simulink model "xEMU_SimulationModel3_rule1"  (R2017b)
settings: Solver=ode4  StartTime=0.0  StopTime=8192  FixedStep=0.01  RelTol=1e-3
undefined symbols (not defined in the file): a1, a2, a3, a4, ACO, BAT, Battery, DCT, DRT, EMS, ENV, Fahrzyklus_VS_modell, height_BAT, leistung, lib_bat, Maximum, Maximum_position, Num_cells, P_FC_max_long, P_FC_min_long, P_FC_step_max, Pbat_charge_max, Pbat_discharge_max, Pfc_max, Pfc_min, SOC_tar, time_peaks, TRM, velocity_peaks
libraries: simulink x5
(part 8 of 15)

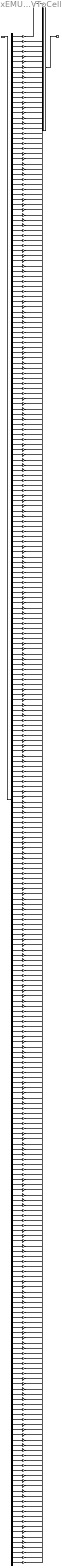
== system xEMU_SimulationModel3_rule1/Battery (BAT)_mittel_02/Cell/Thermal/FVToCell ==
  T_FV : Inport
  AddCell1 : Sum  Inputs=<binary blob, 300 chars, not shown>
  Demux : Demux  Outputs=300
  T_FV_{1..300} (300 alike) : Gain  Gain=0.0033333  SaturateOnIntegerOverflow=on  OutDataTypeStr=Inherit: Same as input  ParamDataTypeStr=Inherit: Same as input
  tag scope: T_CellElement1=global
  wires:
  T_FV/1 -> Demux/1
  Demux/1 -> T_FV_1/1
  Demux/2 -> T_FV_2/1
  Demux/3 -> T_FV_3/1
  Demux/4 -> T_FV_4/1
  Demux/5 -> T_FV_5/1
  Demux/6 -> T_FV_6/1
  Demux/7 -> T_FV_7/1
  Demux/8 -> T_FV_8/1
  Demux/9 -> T_FV_9/1
  Demux/10 -> T_FV_10/1
  Demux/11 -> T_FV_11/1
  Demux/12 -> T_FV_12/1
  Demux/13 -> T_FV_13/1
  Demux/14 -> T_FV_14/1
  Demux/15 -> T_FV_15/1
  Demux/16 -> T_FV_16/1
  Demux/17 -> T_FV_17/1
  Demux/18 -> T_FV_18/1
  Demux/19 -> T_FV_19/1
  Demux/20 -> T_FV_20/1
  Demux/21 -> T_FV_21/1
  Demux/22 -> T_FV_22/1
  Demux/23 -> T_FV_23/1
  Demux/24 -> T_FV_24/1
  Demux/25 -> T_FV_25/1
  Demux/26 -> T_FV_26/1
  Demux/27 -> T_FV_27/1
  Demux/28 -> T_FV_28/1
  Demux/29 -> T_FV_29/1
  Demux/30 -> T_FV_30/1
  Demux/31 -> T_FV_31/1
  Demux/32 -> T_FV_32/1
  Demux/33 -> T_FV_33/1
  Demux/34 -> T_FV_34/1
  Demux/35 -> T_FV_35/1
  Demux/36 -> T_FV_36/1
  Demux/37 -> T_FV_37/1
  Demux/38 -> T_FV_38/1
  Demux/39 -> T_FV_39/1
  Demux/40 -> T_FV_40/1
  Demux/41 -> T_FV_41/1
  Demux/42 -> T_FV_42/1
  Demux/43 -> T_FV_43/1
  Demux/44 -> T_FV_44/1
  Demux/45 -> T_FV_45/1
  Demux/46 -> T_FV_46/1
  Demux/47 -> T_FV_47/1
  Demux/48 -> T_FV_48/1
  Demux/49 -> T_FV_49/1
  Demux/50 -> T_FV_50/1
  Demux/51 -> T_FV_51/1
  Demux/52 -> T_FV_52/1
  Demux/53 -> T_FV_53/1
  Demux/54 -> T_FV_54/1
  Demux/55 -> T_FV_55/1
  Demux/56 -> T_FV_56/1
  Demux/57 -> T_FV_57/1
  Demux/58 -> T_FV_58/1
  Demux/59 -> T_FV_59/1
  Demux/60 -> T_FV_60/1
  Demux/61 -> T_FV_61/1
  Demux/62 -> T_FV_62/1
  Demux/63 -> T_FV_63/1
  Demux/64 -> T_FV_64/1
  Demux/65 -> T_FV_65/1
  Demux/66 -> T_FV_66/1
  Demux/67 -> T_FV_67/1
  Demux/68 -> T_FV_68/1
  Demux/69 -> T_FV_69/1
  Demux/70 -> T_FV_70/1
  Demux/71 -> T_FV_71/1
  Demux/72 -> T_FV_72/1
  Demux/73 -> T_FV_73/1
  Demux/74 -> T_FV_74/1
  Demux/75 -> T_FV_75/1
  Demux/76 -> T_FV_76/1
  Demux/77 -> T_FV_77/1
  Demux/78 -> T_FV_78/1
  Demux/79 -> T_FV_79/1
  Demux/80 -> T_FV_80/1
  Demux/81 -> T_FV_81/1
  Demux/82 -> T_FV_82/1
  Demux/83 -> T_FV_83/1
  Demux/84 -> T_FV_84/1
  Demux/85 -> T_FV_85/1
  Demux/86 -> T_FV_86/1
  Demux/87 -> T_FV_87/1
  Demux/88 -> T_FV_88/1
  Demux/89 -> T_FV_89/1
  Demux/90 -> T_FV_90/1
  Demux/91 -> T_FV_91/1
  Demux/92 -> T_FV_92/1
  Demux/93 -> T_FV_93/1
  Demux/94 -> T_FV_94/1
  Demux/95 -> T_FV_95/1
  Demux/96 -> T_FV_96/1
  Demux/97 -> T_FV_97/1
  Demux/98 -> T_FV_98/1
  Demux/99 -> T_FV_99/1
  Demux/100 -> T_FV_100/1
  Demux/101 -> T_FV_101/1
  Demux/102 -> T_FV_102/1
  Demux/103 -> T_FV_103/1
  Demux/104 -> T_FV_104/1
  Demux/105 -> T_FV_105/1
  Demux/106 -> T_FV_106/1
  Demux/107 -> T_FV_107/1
  Demux/108 -> T_FV_108/1
  Demux/109 -> T_FV_109/1
  Demux/110 -> T_FV_110/1
  Demux/111 -> T_FV_111/1
  Demux/112 -> T_FV_112/1
  Demux/113 -> T_FV_113/1
  Demux/114 -> T_FV_114/1
  Demux/115 -> T_FV_115/1
  Demux/116 -> T_FV_116/1
  Demux/117 -> T_FV_117/1
  Demux/118 -> T_FV_118/1
  Demux/119 -> T_FV_119/1
  Demux/120 -> T_FV_120/1
  Demux/121 -> T_FV_121/1
  Demux/122 -> T_FV_122/1
  Demux/123 -> T_FV_123/1
  Demux/124 -> T_FV_124/1
  Demux/125 -> T_FV_125/1
  Demux/126 -> T_FV_126/1
  Demux/127 -> T_FV_127/1
  Demux/128 -> T_FV_128/1
  Demux/129 -> T_FV_129/1
  Demux/130 -> T_FV_130/1
  Demux/131 -> T_FV_131/1
  Demux/132 -> T_FV_132/1
  Demux/133 -> T_FV_133/1
  Demux/134 -> T_FV_134/1
  Demux/135 -> T_FV_135/1
  Demux/136 -> T_FV_136/1
  Demux/137 -> T_FV_137/1
  Demux/138 -> T_FV_138/1
  Demux/139 -> T_FV_139/1
  Demux/140 -> T_FV_140/1
  Demux/141 -> T_FV_141/1
  Demux/142 -> T_FV_142/1
  Demux/143 -> T_FV_143/1
  Demux/144 -> T_FV_144/1
  Demux/145 -> T_FV_145/1
  Demux/146 -> T_FV_146/1
  Demux/147 -> T_FV_147/1
  Demux/148 -> T_FV_148/1
  Demux/149 -> T_FV_149/1
  Demux/150 -> T_FV_150/1
  Demux/151 -> T_FV_151/1
  Demux/152 -> T_FV_152/1
  Demux/153 -> T_FV_153/1
  Demux/154 -> T_FV_154/1
  Demux/155 -> T_FV_155/1
  Demux/156 -> T_FV_156/1
  Demux/157 -> T_FV_157/1
  Demux/158 -> T_FV_158/1
  Demux/159 -> T_FV_159/1
  Demux/160 -> T_FV_160/1
  Demux/161 -> T_FV_161/1
  Demux/162 -> T_FV_162/1
  Demux/163 -> T_FV_163/1
  Demux/164 -> T_FV_164/1
  Demux/165 -> T_FV_165/1
  Demux/166 -> T_FV_166/1
  Demux/167 -> T_FV_167/1
  Demux/168 -> T_FV_168/1
  Demux/169 -> T_FV_169/1
  Demux/170 -> T_FV_170/1
  Demux/171 -> T_FV_171/1
  Demux/172 -> T_FV_172/1
  Demux/173 -> T_FV_173/1
  Demux/174 -> T_FV_174/1
  Demux/175 -> T_FV_175/1
  Demux/176 -> T_FV_176/1
  Demux/177 -> T_FV_177/1
  Demux/178 -> T_FV_178/1
  Demux/179 -> T_FV_179/1
  Demux/180 -> T_FV_180/1
  Demux/181 -> T_FV_181/1
  Demux/182 -> T_FV_182/1
  Demux/183 -> T_FV_183/1
  Demux/184 -> T_FV_184/1
  Demux/185 -> T_FV_185/1
  Demux/186 -> T_FV_186/1
  Demux/187 -> T_FV_187/1
  Demux/188 -> T_FV_188/1
  Demux/189 -> T_FV_189/1
  Demux/190 -> T_FV_190/1
  Demux/191 -> T_FV_191/1
  Demux/192 -> T_FV_192/1
  Demux/193 -> T_FV_193/1
  Demux/194 -> T_FV_194/1
  Demux/195 -> T_FV_195/1
  Demux/196 -> T_FV_196/1
  Demux/197 -> T_FV_197/1
  Demux/198 -> T_FV_198/1
  Demux/199 -> T_FV_199/1
  Demux/200 -> T_FV_200/1
  Demux/201 -> T_FV_201/1
  Demux/202 -> T_FV_202/1
  Demux/203 -> T_FV_203/1
  Demux/204 -> T_FV_204/1
  Demux/205 -> T_FV_205/1
  Demux/206 -> T_FV_206/1
  Demux/207 -> T_FV_207/1
  Demux/208 -> T_FV_208/1
  Demux/209 -> T_FV_209/1
  Demux/210 -> T_FV_210/1
  Demux/211 -> T_FV_211/1
  Demux/212 -> T_FV_212/1
  Demux/213 -> T_FV_213/1
  Demux/214 -> T_FV_214/1
  Demux/215 -> T_FV_215/1
  Demux/216 -> T_FV_216/1
  Demux/217 -> T_FV_217/1
  Demux/218 -> T_FV_218/1
  Demux/219 -> T_FV_219/1
  Demux/220 -> T_FV_220/1
  Demux/221 -> T_FV_221/1
  Demux/222 -> T_FV_222/1
  Demux/223 -> T_FV_223/1
  Demux/224 -> T_FV_224/1
  Demux/225 -> T_FV_225/1
  Demux/226 -> T_FV_226/1
  Demux/227 -> T_FV_227/1
  Demux/228 -> T_FV_228/1
  Demux/229 -> T_FV_229/1
  Demux/230 -> T_FV_230/1
  Demux/231 -> T_FV_231/1
  Demux/232 -> T_FV_232/1
  Demux/233 -> T_FV_233/1
  Demux/234 -> T_FV_234/1
  Demux/235 -> T_FV_235/1
  Demux/236 -> T_FV_236/1
  Demux/237 -> T_FV_237/1
  Demux/238 -> T_FV_238/1
  Demux/239 -> T_FV_239/1
  Demux/240 -> T_FV_240/1
  Demux/241 -> T_FV_241/1
  Demux/242 -> T_FV_242/1
  Demux/243 -> T_FV_243/1
  Demux/244 -> T_FV_244/1
  Demux/245 -> T_FV_245/1
  Demux/246 -> T_FV_246/1
  Demux/247 -> T_FV_247/1
  Demux/248 -> T_FV_248/1
  Demux/249 -> T_FV_249/1
  Demux/250 -> T_FV_250/1
  Demux/251 -> T_FV_251/1
  Demux/252 -> T_FV_252/1
  Demux/253 -> T_FV_253/1
  Demux/254 -> T_FV_254/1
  Demux/255 -> T_FV_255/1
  Demux/256 -> T_FV_256/1
  Demux/257 -> T_FV_257/1
  Demux/258 -> T_FV_258/1
  Demux/259 -> T_FV_259/1
  Demux/260 -> T_FV_260/1
  Demux/261 -> T_FV_261/1
  Demux/262 -> T_FV_262/1
  Demux/263 -> T_FV_263/1
  Demux/264 -> T_FV_264/1
  Demux/265 -> T_FV_265/1
  Demux/266 -> T_FV_266/1
  Demux/267 -> T_FV_267/1
  Demux/268 -> T_FV_268/1
  Demux/269 -> T_FV_269/1
  Demux/270 -> T_FV_270/1
  Demux/271 -> T_FV_271/1
  Demux/272 -> T_FV_272/1
  Demux/273 -> T_FV_273/1
  Demux/274 -> T_FV_274/1
  Demux/275 -> T_FV_275/1
  Demux/276 -> T_FV_276/1
  Demux/277 -> T_FV_277/1
  Demux/278 -> T_FV_278/1
  Demux/279 -> T_FV_279/1
  Demux/280 -> T_FV_280/1
  Demux/281 -> T_FV_281/1
  Demux/282 -> T_FV_282/1
  Demux/283 -> T_FV_283/1
  Demux/284 -> T_FV_284/1
  Demux/285 -> T_FV_285/1
  Demux/286 -> T_FV_286/1
  Demux/287 -> T_FV_287/1
  Demux/288 -> T_FV_288/1
  Demux/289 -> T_FV_289/1
  Demux/290 -> T_FV_290/1
  Demux/291 -> T_FV_291/1
  Demux/292 -> T_FV_292/1
  Demux/293 -> T_FV_293/1
  Demux/294 -> T_FV_294/1
  Demux/295 -> T_FV_295/1
  Demux/296 -> T_FV_296/1
  Demux/297 -> T_FV_297/1
  Demux/298 -> T_FV_298/1
  Demux/299 -> T_FV_299/1
  Demux/300 -> T_FV_300/1
  AddCell1/1 -> [T_CellElement1]
  T_FV_1/1 -> AddCell1/1
  T_FV_2/1 -> AddCell1/2
  T_FV_3/1 -> AddCell1/3
  T_FV_4/1 -> AddCell1/4
  T_FV_5/1 -> AddCell1/5
  T_FV_6/1 -> AddCell1/6
  T_FV_7/1 -> AddCell1/7
  T_FV_8/1 -> AddCell1/8
  T_FV_9/1 -> AddCell1/9
  T_FV_10/1 -> AddCell1/10
  T_FV_11/1 -> AddCell1/11
  T_FV_12/1 -> AddCell1/12
  T_FV_13/1 -> AddCell1/13
  T_FV_14/1 -> AddCell1/14
  T_FV_15/1 -> AddCell1/15
  T_FV_16/1 -> AddCell1/16
  T_FV_17/1 -> AddCell1/17
  T_FV_18/1 -> AddCell1/18
  T_FV_19/1 -> AddCell1/19
  T_FV_20/1 -> AddCell1/20
  T_FV_21/1 -> AddCell1/21
  T_FV_22/1 -> AddCell1/22
  T_FV_23/1 -> AddCell1/23
  T_FV_24/1 -> AddCell1/24
  T_FV_25/1 -> AddCell1/25
  T_FV_26/1 -> AddCell1/26
  T_FV_27/1 -> AddCell1/27
  T_FV_28/1 -> AddCell1/28
  T_FV_29/1 -> AddCell1/29
  T_FV_30/1 -> AddCell1/30
  T_FV_31/1 -> AddCell1/31
  T_FV_32/1 -> AddCell1/32
  T_FV_33/1 -> AddCell1/33
  T_FV_34/1 -> AddCell1/34
  T_FV_35/1 -> AddCell1/35
  T_FV_36/1 -> AddCell1/36
  T_FV_37/1 -> AddCell1/37
  T_FV_38/1 -> AddCell1/38
  T_FV_39/1 -> AddCell1/39
  T_FV_40/1 -> AddCell1/40
  T_FV_41/1 -> AddCell1/41
  T_FV_42/1 -> AddCell1/42
  T_FV_43/1 -> AddCell1/43
  T_FV_44/1 -> AddCell1/44
  T_FV_45/1 -> AddCell1/45
  T_FV_46/1 -> AddCell1/46
  T_FV_47/1 -> AddCell1/47
  T_FV_48/1 -> AddCell1/48
  T_FV_49/1 -> AddCell1/49
  T_FV_50/1 -> AddCell1/50
  T_FV_51/1 -> AddCell1/51
  T_FV_52/1 -> AddCell1/52
  T_FV_53/1 -> AddCell1/53
  T_FV_54/1 -> AddCell1/54
  T_FV_55/1 -> AddCell1/55
  T_FV_56/1 -> AddCell1/56
  T_FV_57/1 -> AddCell1/57
  T_FV_58/1 -> AddCell1/58
  T_FV_59/1 -> AddCell1/59
  T_FV_60/1 -> AddCell1/60
  T_FV_61/1 -> AddCell1/61
  T_FV_62/1 -> AddCell1/62
  T_FV_63/1 -> AddCell1/63
  T_FV_64/1 -> AddCell1/64
  T_FV_65/1 -> AddCell1/65
  T_FV_66/1 -> AddCell1/66
  T_FV_67/1 -> AddCell1/67
  T_FV_68/1 -> AddCell1/68
  T_FV_69/1 -> AddCell1/69
  T_FV_70/1 -> AddCell1/70
  T_FV_71/1 -> AddCell1/71
  T_FV_72/1 -> AddCell1/72
  T_FV_73/1 -> AddCell1/73
  T_FV_74/1 -> AddCell1/74
  T_FV_75/1 -> AddCell1/75
  T_FV_76/1 -> AddCell1/76
  T_FV_77/1 -> AddCell1/77
  T_FV_78/1 -> AddCell1/78
  T_FV_79/1 -> AddCell1/79
  T_FV_80/1 -> AddCell1/80
  T_FV_81/1 -> AddCell1/81
  T_FV_82/1 -> AddCell1/82
  T_FV_83/1 -> AddCell1/83
  T_FV_84/1 -> AddCell1/84
  T_FV_85/1 -> AddCell1/85
  T_FV_86/1 -> AddCell1/86
  T_FV_87/1 -> AddCell1/87
  T_FV_88/1 -> AddCell1/88
  T_FV_89/1 -> AddCell1/89
  T_FV_90/1 -> AddCell1/90
  T_FV_91/1 -> AddCell1/91
  T_FV_92/1 -> AddCell1/92
  T_FV_93/1 -> AddCell1/93
  T_FV_94/1 -> AddCell1/94
  T_FV_95/1 -> AddCell1/95
  T_FV_96/1 -> AddCell1/96
  T_FV_97/1 -> AddCell1/97
  T_FV_98/1 -> AddCell1/98
  T_FV_99/1 -> AddCell1/99
  T_FV_100/1 -> AddCell1/100
  T_FV_101/1 -> AddCell1/101
  T_FV_102/1 -> AddCell1/102
  T_FV_103/1 -> AddCell1/103
  T_FV_104/1 -> AddCell1/104
  T_FV_105/1 -> AddCell1/105
  T_FV_106/1 -> AddCell1/106
  T_FV_107/1 -> AddCell1/107
  T_FV_108/1 -> AddCell1/108
  T_FV_109/1 -> AddCell1/109
  T_FV_110/1 -> AddCell1/110
  T_FV_111/1 -> AddCell1/111
  T_FV_112/1 -> AddCell1/112
  T_FV_113/1 -> AddCell1/113
  T_FV_114/1 -> AddCell1/114
  T_FV_115/1 -> AddCell1/115
  T_FV_116/1 -> AddCell1/116
  T_FV_117/1 -> AddCell1/117
  T_FV_118/1 -> AddCell1/118
  T_FV_119/1 -> AddCell1/119
  T_FV_120/1 -> AddCell1/120
  T_FV_121/1 -> AddCell1/121
  T_FV_122/1 -> AddCell1/122
  T_FV_123/1 -> AddCell1/123
  T_FV_124/1 -> AddCell1/124
  T_FV_125/1 -> AddCell1/125
  T_FV_126/1 -> AddCell1/126
  T_FV_127/1 -> AddCell1/127
  T_FV_128/1 -> AddCell1/128
  T_FV_129/1 -> AddCell1/129
  T_FV_130/1 -> AddCell1/130
  T_FV_131/1 -> AddCell1/131
  T_FV_132/1 -> AddCell1/132
  T_FV_133/1 -> AddCell1/133
  T_FV_134/1 -> AddCell1/134
  T_FV_135/1 -> AddCell1/135
  T_FV_136/1 -> AddCell1/136
  T_FV_137/1 -> AddCell1/137
  T_FV_138/1 -> AddCell1/138
  T_FV_139/1 -> AddCell1/139
  T_FV_140/1 -> AddCell1/140
  T_FV_141/1 -> AddCell1/141
  T_FV_142/1 -> AddCell1/142
  T_FV_143/1 -> AddCell1/143
  T_FV_144/1 -> AddCell1/144
  T_FV_145/1 -> AddCell1/145
  T_FV_146/1 -> AddCell1/146
  T_FV_147/1 -> AddCell1/147
  T_FV_148/1 -> AddCell1/148
  T_FV_149/1 -> AddCell1/149
  T_FV_150/1 -> AddCell1/150
  T_FV_151/1 -> AddCell1/151
  T_FV_152/1 -> AddCell1/152
  T_FV_153/1 -> AddCell1/153
  T_FV_154/1 -> AddCell1/154
  T_FV_155/1 -> AddCell1/155
  T_FV_156/1 -> AddCell1/156
  T_FV_157/1 -> AddCell1/157
  T_FV_158/1 -> AddCell1/158
  T_FV_159/1 -> AddCell1/159
  T_FV_160/1 -> AddCell1/160
  T_FV_161/1 -> AddCell1/161
  T_FV_162/1 -> AddCell1/162
  T_FV_163/1 -> AddCell1/163
  T_FV_164/1 -> AddCell1/164
  T_FV_165/1 -> AddCell1/165
  T_FV_166/1 -> AddCell1/166
  T_FV_167/1 -> AddCell1/167
  T_FV_168/1 -> AddCell1/168
  T_FV_169/1 -> AddCell1/169
  T_FV_170/1 -> AddCell1/170
  T_FV_171/1 -> AddCell1/171
  T_FV_172/1 -> AddCell1/172
  T_FV_173/1 -> AddCell1/173
  T_FV_174/1 -> AddCell1/174
  T_FV_175/1 -> AddCell1/175
  T_FV_176/1 -> AddCell1/176
  T_FV_177/1 -> AddCell1/177
  T_FV_178/1 -> AddCell1/178
  T_FV_179/1 -> AddCell1/179
  T_FV_180/1 -> AddCell1/180
  T_FV_181/1 -> AddCell1/181
  T_FV_182/1 -> AddCell1/182
  T_FV_183/1 -> AddCell1/183
  T_FV_184/1 -> AddCell1/184
  T_FV_185/1 -> AddCell1/185
  T_FV_186/1 -> AddCell1/186
  T_FV_187/1 -> AddCell1/187
  T_FV_188/1 -> AddCell1/188
  T_FV_189/1 -> AddCell1/189
  T_FV_190/1 -> AddCell1/190
  T_FV_191/1 -> AddCell1/191
  T_FV_192/1 -> AddCell1/192
  T_FV_193/1 -> AddCell1/193
  T_FV_194/1 -> AddCell1/194
  T_FV_195/1 -> AddCell1/195
  T_FV_196/1 -> AddCell1/196
  T_FV_197/1 -> AddCell1/197
  T_FV_198/1 -> AddCell1/198
  T_FV_199/1 -> AddCell1/199
  T_FV_200/1 -> AddCell1/200
  T_FV_201/1 -> AddCell1/201
  T_FV_202/1 -> AddCell1/202
  T_FV_203/1 -> AddCell1/203
  T_FV_204/1 -> AddCell1/204
  T_FV_205/1 -> AddCell1/205
  T_FV_206/1 -> AddCell1/206
  T_FV_207/1 -> AddCell1/207
  T_FV_208/1 -> AddCell1/208
  T_FV_209/1 -> AddCell1/209
  T_FV_210/1 -> AddCell1/210
  T_FV_211/1 -> AddCell1/211
  T_FV_212/1 -> AddCell1/212
  T_FV_213/1 -> AddCell1/213
  T_FV_214/1 -> AddCell1/214
  T_FV_215/1 -> AddCell1/215
  T_FV_216/1 -> AddCell1/216
  T_FV_217/1 -> AddCell1/217
  T_FV_218/1 -> AddCell1/218
  T_FV_219/1 -> AddCell1/219
  T_FV_220/1 -> AddCell1/220
  T_FV_221/1 -> AddCell1/221
  T_FV_222/1 -> AddCell1/222
  T_FV_223/1 -> AddCell1/223
  T_FV_224/1 -> AddCell1/224
  T_FV_225/1 -> AddCell1/225
  T_FV_226/1 -> AddCell1/226
  T_FV_227/1 -> AddCell1/227
  T_FV_228/1 -> AddCell1/228
  T_FV_229/1 -> AddCell1/229
  T_FV_230/1 -> AddCell1/230
  T_FV_231/1 -> AddCell1/231
  T_FV_232/1 -> AddCell1/232
  T_FV_233/1 -> AddCell1/233
  T_FV_234/1 -> AddCell1/234
  T_FV_235/1 -> AddCell1/235
  T_FV_236/1 -> AddCell1/236
  T_FV_237/1 -> AddCell1/237
  T_FV_238/1 -> AddCell1/238
  T_FV_239/1 -> AddCell1/239
  T_FV_240/1 -> AddCell1/240
  T_FV_241/1 -> AddCell1/241
  T_FV_242/1 -> AddCell1/242
  T_FV_243/1 -> AddCell1/243
  T_FV_244/1 -> AddCell1/244
  T_FV_245/1 -> AddCell1/245
  T_FV_246/1 -> AddCell1/246
  T_FV_247/1 -> AddCell1/247
  T_FV_248/1 -> AddCell1/248
  T_FV_249/1 -> AddCell1/249
  T_FV_250/1 -> AddCell1/250
  T_FV_251/1 -> AddCell1/251
  T_FV_252/1 -> AddCell1/252
  T_FV_253/1 -> AddCell1/253
  T_FV_254/1 -> AddCell1/254
  T_FV_255/1 -> AddCell1/255
  T_FV_256/1 -> AddCell1/256
  T_FV_257/1 -> AddCell1/257
  T_FV_258/1 -> AddCell1/258
  T_FV_259/1 -> AddCell1/259
  T_FV_260/1 -> AddCell1/260
  T_FV_261/1 -> AddCell1/261
  T_FV_262/1 -> AddCell1/262
  T_FV_263/1 -> AddCell1/263
  T_FV_264/1 -> AddCell1/264
  T_FV_265/1 -> AddCell1/265
  T_FV_266/1 -> AddCell1/266
  T_FV_267/1 -> AddCell1/267
  T_FV_268/1 -> AddCell1/268
  T_FV_269/1 -> AddCell1/269
  T_FV_270/1 -> AddCell1/270
  T_FV_271/1 -> AddCell1/271
  T_FV_272/1 -> AddCell1/272
  T_FV_273/1 -> AddCell1/273
  T_FV_274/1 -> AddCell1/274
  T_FV_275/1 -> AddCell1/275
  T_FV_276/1 -> AddCell1/276
  T_FV_277/1 -> AddCell1/277
  T_FV_278/1 -> AddCell1/278
  T_FV_279/1 -> AddCell1/279
  T_FV_280/1 -> AddCell1/280
  T_FV_281/1 -> AddCell1/281
  T_FV_282/1 -> AddCell1/282
  T_FV_283/1 -> AddCell1/283
  T_FV_284/1 -> AddCell1/284
  T_FV_285/1 -> AddCell1/285
  T_FV_286/1 -> AddCell1/286
  T_FV_287/1 -> AddCell1/287
  T_FV_288/1 -> AddCell1/288
  T_FV_289/1 -> AddCell1/289
  T_FV_290/1 -> AddCell1/290
  T_FV_291/1 -> AddCell1/291
  T_FV_292/1 -> AddCell1/292
  T_FV_293/1 -> AddCell1/293
  T_FV_294/1 -> AddCell1/294
  T_FV_295/1 -> AddCell1/295
  T_FV_296/1 -> AddCell1/296
  T_FV_297/1 -> AddCell1/297
  T_FV_298/1 -> AddCell1/298
  T_FV_299/1 -> AddCell1/299
  T_FV_300/1 -> AddCell1/300

== system xEMU_SimulationModel3_rule1/Battery (BAT)_mittel_02/Cell/TotalValues/Component0 ==
  ColConst : Constant  Value=0
  RowConst : Constant  Value=0
  Row : Outport
  Col : Outport  Port=2
  Value : Outport  Port=3
  wires:
  ColConst/1 -> Col/1
  RowConst/1 -> Row/1
  [InputCurrent] -> Value/1

== system xEMU_SimulationModel3_rule1/Battery (BAT)_mittel_02/Cell/TotalValues/Component1 ==
  Add2_1 : Sum
  Add3_1 : Sum
  Add3_2 : Sum
  Add4_1 : Sum
  ColConst : Constant  Value=0
  Mul2_3 : Product
  RowConst : Constant
  Row : Outport
  Col : Outport  Port=2
  Value : Outport  Port=3
  wires:
  ColConst/1 -> Col/1
  RowConst/1 -> Row/1
  Add4_1/1 -> Value/1
  Add3_1/1 -> Add4_1/1
  Add2_1/1 -> Add3_1/1
  [State1] -> Add2_1/1
  [State2] -> Add2_1/2
  [State3] -> Add3_1/2
  Add3_2/1 -> Add4_1/2
  Mul2_3/1 -> Add3_2/1
  [InputCurrent] -> Mul2_3/1
  [ID2_ObjR] -> Mul2_3/2
  [ID6_ObjV] -> Add3_2/2

== system xEMU_SimulationModel3_rule1/Battery (BAT)_mittel_02/Cell/TotalValues/Component2 ==
  Add4_1 : Sum
  Add5_1 : Sum
  Add6_1 : Sum
  ColConst : Constant  Value=0
  Div3_1 : Product  Inputs=*/
  Div3_2 : Product  Inputs=*/
  Div4_2 : Product  Inputs=*/
  Mul5_2 : Product
  RowConst : Constant  Value=2
  Squ2_1 : Math  Operator=square  SaturateOnIntegerOverflow=on
  Squ2_3 : Math  Operator=square  SaturateOnIntegerOverflow=on
  Squ3_3 : Math  Operator=square  SaturateOnIntegerOverflow=on
  Squ4_3 : Math  Operator=square  SaturateOnIntegerOverflow=on
  Row : Outport
  Col : Outport  Port=2
  Value : Outport  Port=3
  wires:
  ColConst/1 -> Col/1
  RowConst/1 -> Row/1
  Add6_1/1 -> Value/1
  Add5_1/1 -> Add6_1/1
  Add4_1/1 -> Add5_1/1
  Div3_1/1 -> Add4_1/1
  Squ2_1/1 -> Div3_1/1
  [State1] -> Squ2_1/1
  [ID3_ObjR] -> Div3_1/2
  Div3_2/1 -> Add4_1/2
  Squ2_3/1 -> Div3_2/1
  [State2] -> Squ2_3/1
  [ID4_ObjR] -> Div3_2/2
  Div4_2/1 -> Add5_1/2
  Squ3_3/1 -> Div4_2/1
  [State3] -> Squ3_3/1
  [ID5_ObjR] -> Div4_2/2
  Mul5_2/1 -> Add6_1/2
  Squ4_3/1 -> Mul5_2/1
  [InputCurrent] -> Squ4_3/1
  [ID2_ObjR] -> Mul5_2/2

== system xEMU_SimulationModel3_rule1/Drive Train (DRT)/Converter and traction motor/traction_motor_kennfeldbasiert/Subsystem ==
  M : Inport
  "lookuptable_Pv " : Inport  Port=2
  "n " : Inport  Port=3
  MATLAB Function : MATLAB Function  TreatAsAtomicUnit=on
  n-D Lookup Pv_obergrenze : Lookup_n-D  NumberOfTableDimensions=1  BreakpointsForDimension1=speedvector  BreakpointsForDimension3=[5, 7]  Table=Pv_obergrenze  InternalRulePriority=Speed  RndMeth=Simplest  InputSameDT=on
  n-D Lookup Pv_untergrenze : Lookup_n-D  NumberOfTableDimensions=1  BreakpointsForDimension1=speedvector  BreakpointsForDimension3=[5, 7]  Table=Pv_untergrenze  InternalRulePriority=Speed  RndMeth=Simplest  InputSameDT=on
  Pv_motor : Outport
  wires:
  "n "/1 -> n-D Lookup Pv_untergrenze/1, n-D Lookup Pv_obergrenze/1
  M/1 -> MATLAB Function/4(M)
  n-D Lookup Pv_untergrenze/1 -> MATLAB Function/3(Pv_min)
  n-D Lookup Pv_obergrenze/1 -> MATLAB Function/2(Pv_max)
  "lookuptable_Pv "/1 -> MATLAB Function/1(Pv)
  MATLAB Function/1(y) -> Pv_motor/1

== system xEMU_SimulationModel3_rule1/Drive Train (DRT)/Converter and traction motor/traction_motor_kennfeldbasiert/Subsystem1 ==
  M : Inport
  "lookuptable_coshpi " : Inport  Port=2
  "n " : Inport  Port=3
  MATLAB Function : MATLAB Function  TreatAsAtomicUnit=on
  n-D Lookup Pv_obergrenze : Lookup_n-D  NumberOfTableDimensions=1  BreakpointsForDimension1=speedvector  BreakpointsForDimension3=[5, 7]  Table=cosphi_obergrenze  InternalRulePriority=Speed  RndMeth=Simplest  InputSameDT=on
  n-D Lookup Pv_untergrenze : Lookup_n-D  NumberOfTableDimensions=1  BreakpointsForDimension1=speedvector  BreakpointsForDimension3=[5, 7]  Table=cosphi_untergrenze  InternalRulePriority=Speed  RndMeth=Simplest  InputSameDT=on
  coshpi_motor : Outport
  wires:
  "n "/1 -> n-D Lookup Pv_untergrenze/1, n-D Lookup Pv_obergrenze/1
  M/1 -> MATLAB Function/4(M)
  n-D Lookup Pv_untergrenze/1 -> MATLAB Function/3(cosphi_min)
  n-D Lookup Pv_obergrenze/1 -> MATLAB Function/2(cosphi_max)
  "lookuptable_coshpi "/1 -> MATLAB Function/1(cosphi)
  MATLAB Function/1(y) -> coshpi_motor/1

== system xEMU_SimulationModel3_rule1/Drive Train (DRT)/Converter and traction motor/traction_motor_kennfeldbasiert/Subsystem2 ==
  M : Inport
  "lookuptable_coshpi " : Inport  Port=2
  "n " : Inport  Port=3
  MATLAB Function : MATLAB Function  TreatAsAtomicUnit=on
  n-D Lookup Pv_obergrenze : Lookup_n-D  NumberOfTableDimensions=1  BreakpointsForDimension1=speedvector  BreakpointsForDimension3=[5, 7]  Table=U_LL_obergrenze  InternalRulePriority=Speed  RndMeth=Simplest  InputSameDT=on
  n-D Lookup Pv_untergrenze : Lookup_n-D  NumberOfTableDimensions=1  BreakpointsForDimension1=speedvector  BreakpointsForDimension3=[5, 7]  Table=U_LL_untergrenze  InternalRulePriority=Speed  RndMeth=Simplest  InputSameDT=on
  U_LL_motor : Outport
  wires:
  "n "/1 -> n-D Lookup Pv_untergrenze/1, n-D Lookup Pv_obergrenze/1
  M/1 -> MATLAB Function/4(M)
  n-D Lookup Pv_untergrenze/1 -> MATLAB Function/3(U_LL_min)
  n-D Lookup Pv_obergrenze/1 -> MATLAB Function/2(U_LL_max)
  "lookuptable_coshpi "/1 -> MATLAB Function/1(U_LL)
  MATLAB Function/1(y) -> U_LL_motor/1

== system xEMU_SimulationModel3_rule1/Drive Train (DRT)/Converter and traction motor/traction_motor_kennfeldbasiert/Subsystem3 ==
  M : Inport
  "lookuptable_coshpi " : Inport  Port=2
  "n " : Inport  Port=3
  MATLAB Function : MATLAB Function  TreatAsAtomicUnit=on
  n-D Lookup Pv_obergrenze : Lookup_n-D  NumberOfTableDimensions=1  BreakpointsForDimension1=speedvector  BreakpointsForDimension3=[5, 7]  Table=I_strang_obergrenze  InternalRulePriority=Speed  RndMeth=Simplest  InputSameDT=on
  n-D Lookup Pv_untergrenze : Lookup_n-D  NumberOfTableDimensions=1  BreakpointsForDimension1=speedvector  BreakpointsForDimension3=[5, 7]  Table=I_strang_untergrenze  InternalRulePriority=Speed  RndMeth=Simplest  InputSameDT=on
  I_strang_motor : Outport
  wires:
  "n "/1 -> n-D Lookup Pv_untergrenze/1, n-D Lookup Pv_obergrenze/1
  M/1 -> MATLAB Function/4(M)
  n-D Lookup Pv_untergrenze/1 -> MATLAB Function/3(I_strang_min)
  n-D Lookup Pv_obergrenze/1 -> MATLAB Function/2(I_strang_max)
  "lookuptable_coshpi "/1 -> MATLAB Function/1(I_strang)
  MATLAB Function/1(y) -> I_strang_motor/1

== system xEMU_SimulationModel3_rule1/Drive Train (DRT)/Slipmodel and Traction /Variant Subsystem1/Mit_Schlupf_nach_Kalker ==
  T_EMAdemandper_axis_Nm : Inport
  v_train_m/s : Inport  Port=2
  adhesionCoefficient_abs : Inport  Port=3
  Resistance of tire : Inport  Port=4
  Fz_tire : Inport  Port=5
  Gain3 : Gain  Gain=2
  Slip Model : Subsystem
  Tire Dynamics : Subsystem
  F_traction_peraxis_N : Outport
  WheelSpeed_rad/s : Outport  Port=2
  f_traction_tire : Outport  Port=3
  wires:
  Resistance of tire/1 -> Tire Dynamics/1(Resistance of tire)
  T_EMAdemandper_axis_Nm/1 -> Tire Dynamics/2(T_EMAdemandper_axis_Nm)
  v_train_m/s/1 -> Tire Dynamics/3(v_train_m/s)
  adhesionCoefficient_abs/1 -> Slip Model/3(adhesion)
  Tire Dynamics/2(WheelSpeed_rad/s) -> WheelSpeed_rad/s/1
  Tire Dynamics/1(slip) -> Slip Model/2(slip)
  Fz_tire/1 -> Slip Model/1(Fz_tire)
  Slip Model/1(f_traction_tire) -> Gain3/1, f_traction_tire/1
  Gain3/1 -> F_traction_peraxis_N/1

== system xEMU_SimulationModel3_rule1/Drive Train (DRT)/Slipmodel and Traction /Variant Subsystem1/Mit_Schlupf_nach_Yoshiki ==
  T_EMAdemandper_axis_Nm : Inport
  v_train_m/s : Inport  Port=2
  Resistance of tire : Inport  Port=3
  Fz_tire : Inport  Port=4
  adhesionCoefficient_abs : Inport  Port=5
  Gain3 : Gain  Gain=2
  Slip Model : Subsystem
  Tire Dynamics : Subsystem
  F_traction_peraxis_N : Outport
  WheelSpeed_rad/s : Outport  Port=2
  f_traction_tire : Outport  Port=3
  wires:
  Resistance of tire/1 -> Tire Dynamics/1(Resistance of tire)
  Fz_tire/1 -> Slip Model/1(Fz_tire)
  Tire Dynamics/1(slip_speed) -> Slip Model/2(slip_speed)
  Tire Dynamics/2(WheelSpeed_rad/s) -> Slip Model/4(wheelspeed), WheelSpeed_rad/s/1
  Gain3/1 -> F_traction_peraxis_N/1
  Slip Model/1(f_traction_tire) -> f_traction_tire/1, Gain3/1
  T_EMAdemandper_axis_Nm/1 -> Tire Dynamics/2(T_EMAdemandper_axis_Nm)
  v_train_m/s/1 -> Tire Dynamics/3(v_train_m/s)
  adhesionCoefficient_abs/1 -> Slip Model/3(adhesionCoefficient_abs)

== system xEMU_SimulationModel3_rule1/Drive Train (DRT)/Slipmodel and Traction /Variant Subsystem1/Ohne_Schlupf ==
  T_EMAdemandper_axis_Nm : Inport
  v_train_m/s : Inport  Port=2
  Gain2 : Gain  Gain=1/R_wheel_drt_m
  Gain4 : Gain  Gain=1/R_wheel_drt_m
  F_traction_peraxis_N : Outport
  WheelSpeed_rad/s : Outport  Port=2
  wires:
  Gain4/1 -> F_traction_peraxis_N/1
  Gain2/1 -> WheelSpeed_rad/s/1
  v_train_m/s/1 -> Gain2/1
  T_EMAdemandper_axis_Nm/1 -> Gain4/1

== system xEMU_SimulationModel3_rule1/Energy Manager (EMA)/Kern von EMS/P_load_aver/Subsystem ==
  F_EMAdemand_N : Inport
  Gradient_force : Inport  Port=2
  n_motor_rpm : Inport  Port=3
  Add1 : Sum
  Divide3 : Product  Inputs=*/
  Gain3 : Gain  Gain=DRT.slipmodel.R_wheel_drt_m/DRT.motor.gearratio_drt
  Product5 : Product
  Sum : Sum  Inputs=|+++
  dcdc efficiency : MATLAB Function  TreatAsAtomicUnit=on
  traction_motor_kennfeldbasiert : Subsystem
  korrigierte_Pload : Outport
  wires:
  Add1/1 -> Gain3/1  "corrected force"
  Gradient_force/1 -> Add1/2
  [num_EM] -> Product5/1
  F_EMAdemand_N/1 -> Add1/1
  traction_motor_kennfeldbasiert/1("P_el_corr ") -> Product5/2  "corrected Pel per motor"
  [P_apu] -> Sum/3
  Product5/1 -> Sum/1
  Sum/1 -> dcdc efficiency/1(u)
  Divide3/1 -> traction_motor_kennfeldbasiert/1("M_corr ")  "corrected M"
  Gain3/1 -> Divide3/1
  [P_clima] -> Sum/2
  n_motor_rpm/1 -> traction_motor_kennfeldbasiert/2(n)
  dcdc efficiency/1(y) -> korrigierte_Pload/1
  [num_EM] -> Divide3/2

== system xEMU_SimulationModel3_rule1/Train Dynamics (TRM)/Variant Subsystem/v_s_model/Driver1 ==
  v_drivingCycle_m/s : Inport
  v_train : Inport  Port=2
  MATLAB Function : MATLAB Function  TreatAsAtomicUnit=on
  MATLAB Function1 : MATLAB Function  Commented=on  TreatAsAtomicUnit=on
  PID Controller1 : simulink/Continuous/PID Controller  Controller=PID  TimeDomain=Continuous-time  SampleTime=-1  IntegratorMethod=Forward Euler  FilterMethod=Forward Euler  Form=Parallel  UseFilter=on  ControllerParametersSource=internal  P=50  I=2  D=0  N=100  InitialConditionSource=internal  InitialConditionForIntegrator=0  InitialConditionForFilter=0  ExternalReset=falling  LimitOutput=on  UpperSaturationLimit=100  LowerSaturationLimit=-100  LinearizeAsGain=on  AntiWindupMode=clamping  Kb=1  TrackingMode=off  Kt=1  PParamMin=[]  PParamMax=[]  IParamMin=[]  IParamMax=[]  DParamMin=[]  DParamMax=[]  NParamMin=[]  NParamMax=[]  KbParamMin=[]  KbParamMax=[]  KtParamMin=[]  KtParamMax=[]  POutMin=[]  POutMax=[]  IOutMin=[]  IOutMax=[]  DOutMin=[]  DOutMax=[]  NOutMin=[]  NOutMax=[]  KbOutMin=[]  KbOutMax=[]  KtOutMin=[]  KtOutMax=[]  IntegratorOutMin=[]  IntegratorOutMax=[]  FilterOutMin=[]  FilterOutMax=[]  SumOutMin=[]  SumOutMax=[]  SumI1OutMin=[]  SumI1OutMax=[]  SumI2OutMin=[]  SumI2OutMax=[]  SumI3OutMin=[]  SumI3OutMax=[]  SumDOutMin=[]  SumDOutMax=[]  SaturationOutMin=[]  SaturationOutMax=[]  IntegratorContinuousStateAttributes=''  IntegratorStateMustResolveToSignalObject=off  IntegratorRTWStateStorageClass=Auto  FilterContinuousStateAttributes=''  FilterStateMustResolveToSignalObject=off  FilterRTWStateStorageClass=Auto  DifferentiatorICPrevScaledInput=0  DifferentiatorOutMin=[]  DifferentiatorOutMax=[]  InitialConditionSetting=State (most efficient)  FilterDiffOutCoefMin=[]  FilterDiffOutCoefMax=[]  SumDenOutMin=[]  SumDenOutMax=[]  SumNumOutMin=[]  SumNumOutMax=[]  ReciprocalOutMin=[]  ReciprocalOutMax=[]  DivideOutMin=[]  DivideOutMax=[]  TunerSelectOption=Transfer Function Based (PID Tuner App)
  Scope : Scope
  Scope1 : Scope
  Sum2 : Sum  Inputs=|+-
  F_tractionDemand_N : Outport
  wires:
  v_drivingCycle_m/s/1 -> Sum2/1, MATLAB Function1/1(vsoll)
  Sum2/1 -> MATLAB Function1/2(dv), PID Controller1/1
  v_train/1 -> Sum2/2
  MATLAB Function1/1(Reset) -> PID Controller1/2
  PID Controller1/1 -> Scope/1, MATLAB Function/1(pid)
  MATLAB Function/1(s) -> Scope1/1, F_tractionDemand_N/1

== system xEMU_SimulationModel3_rule1/Train Dynamics (TRM)/Variant Subsystem/v_s_model/Driving Resistances ==
  v_train : Inport
  total mass : Inport  Port=2
  gradient : Inport  Port=3
  Gain : Gain  Gain=g_drt
  Gain1 : Gain  Gain=0.0015
  Gain2 : Gain  Gain=1/1000*3.6*0.025
  MATLAB Function1 : MATLAB Function  TreatAsAtomicUnit=on
  Product : Product
  Product1 : Product
  Product2 : Product
  Subtract : Sum  Inputs=++++
  Trigonometric Function : Trigonometry
  Trigonometric Function2 : Trigonometry  Operator=cos
  air resistance : Fcn  Expr=Cw_tdn_abs*A_tdn_m2*(PI_tdn/2)*(u)^2
  Fahrwiderstand_N : Outport
  wires:
  Subtract/1 -> Fahrwiderstand_N/1
  Product/1 -> Subtract/3
  air resistance/1 -> Subtract/2
  Trigonometric Function/1 -> Product/1
  Gain1/1 -> Product2/1
  Product2/1 -> MATLAB Function1/2(froll)
  Trigonometric Function2/1 -> Product2/2
  gradient/1 -> Trigonometric Function2/1, Trigonometric Function/1
  Gain/1 -> Gain1/1, Product/2
  MATLAB Function1/1(Froll) -> Subtract/4
  v_train/1 -> Product1/1, MATLAB Function1/1(v), air resistance/1
  total mass/1 -> Product1/2, Gain/1
  Gain2/1 -> Subtract/1
  Product1/1 -> Gain2/1

== system xEMU_SimulationModel3_rule1/Train Dynamics (TRM)/Variant Subsystem/v_s_model/Train Longitudinal Dynamics ==
  note: a
  n_passengers_abs : Inport
  F_traction_N : Inport  Port=2
  Fahrwiderstand_N : Inport  Port=3
  Compare To Constant : simulink/Logic and Bit Operations/Compare To Constant  relop=>=  const=1  OutDataTypeStr=boolean
  Constant : Constant  Value=m_train_tdn_kg
  Constant1 : Constant
  Constant2 : Constant  Value=max(Fahrzyklus_VS_modell.Positionm)
  Divide : Product  Inputs=/*
  Divide1 : Product  Inputs=*/
  Gain : Gain  Gain=m_passenger_tdn_kg
  Gain1 : Gain  Gain=1/100
  Integrator : Integrator  LimitOutput=on  LowerSaturationLimit=0
  Integrator1 : Integrator
  Integrator2 : Integrator  ExternalReset=either
  Scope : Scope
  Scope2 : Scope
  Steigung : Lookup_n-D  NumberOfTableDimensions=1  BreakpointsForDimension1=Fahrzyklus_VS_modell.Positionm  Table=Fahrzyklus_VS_modell.Steigung  InternalRulePriority=Speed  RndMeth=Simplest  InputSameDT=on
  Subtract : Sum
  Sum : Sum  Inputs=-+|
  Trigonometric Function : Trigonometry  Operator=atan
  V-Table : Lookup_n-D  NumberOfTableDimensions=1  BreakpointsForDimension1=Fahrzyklus_VS_modell.s  Table=Fahrzyklus_VS_modell.v  InternalRulePriority=Speed  RndMeth=Simplest  InputSameDT=on
  v_soll_m/s : Outport
  v_train_m/s : Outport  Port=2
  total_mass_kg : Outport  Port=3
  Steigung_soll : Outport  Port=4
  wires:
  Fahrwiderstand_N/1 -> Sum/1
  Sum/1 -> Divide/2
  n_passengers_abs/1 -> Gain/1
  Constant/1 -> Subtract/2
  Gain/1 -> Subtract/1
  F_traction_N/1 -> Sum/2
  Divide/1 -> Integrator/1
  Integrator1/1 -> Divide1/1, Scope2/1, Steigung/1, V-Table/1  "s"
  Integrator/1 -> v_train_m/s/1, Integrator1/1  "v_train_m/s"
  Steigung/1 -> Gain1/1
  V-Table/1 -> v_soll_m/s/1
  Gain1/1 -> Trigonometric Function/1
  Trigonometric Function/1 -> Steigung_soll/1
  Constant1/1 -> Integrator2/1
  Constant2/1 -> Divide1/2
  Divide1/1 -> Compare To Constant/1
  Compare To Constant/1 -> Integrator2/2
  Integrator2/1 -> Scope/1
  Subtract/1 -> Divide/1, total_mass_kg/1

== system xEMU_SimulationModel3_rule1/Train Dynamics (TRM)/Variant Subsystem/v_t_model/Driver1 ==
  v_drivingCycle_m/s : Inport
  v_train : Inport  Port=2
  MATLAB Function : MATLAB Function  TreatAsAtomicUnit=on
  PID Controller1 : simulink/Continuous/PID Controller  Controller=PID  TimeDomain=Continuous-time  SampleTime=-1  IntegratorMethod=Forward Euler  FilterMethod=Forward Euler  Form=Parallel  UseFilter=on  ControllerParametersSource=internal  P=500  I=2  D=0  N=100  InitialConditionSource=internal  InitialConditionForIntegrator=0  InitialConditionForFilter=0  ExternalReset=none  LimitOutput=on  UpperSaturationLimit=100  LowerSaturationLimit=-100  LinearizeAsGain=on  AntiWindupMode=clamping  Kb=1  TrackingMode=off  Kt=1  PParamMin=[]  PParamMax=[]  IParamMin=[]  IParamMax=[]  DParamMin=[]  DParamMax=[]  NParamMin=[]  NParamMax=[]  KbParamMin=[]  KbParamMax=[]  KtParamMin=[]  KtParamMax=[]  POutMin=[]  POutMax=[]  IOutMin=[]  IOutMax=[]  DOutMin=[]  DOutMax=[]  NOutMin=[]  NOutMax=[]  KbOutMin=[]  KbOutMax=[]  KtOutMin=[]  KtOutMax=[]  IntegratorOutMin=[]  IntegratorOutMax=[]  FilterOutMin=[]  FilterOutMax=[]  SumOutMin=[]  SumOutMax=[]  SumI1OutMin=[]  SumI1OutMax=[]  SumI2OutMin=[]  SumI2OutMax=[]  SumI3OutMin=[]  SumI3OutMax=[]  SumDOutMin=[]  SumDOutMax=[]  SaturationOutMin=[]  SaturationOutMax=[]  IntegratorContinuousStateAttributes=''  IntegratorStateMustResolveToSignalObject=off  IntegratorRTWStateStorageClass=Auto  FilterContinuousStateAttributes=''  FilterStateMustResolveToSignalObject=off  FilterRTWStateStorageClass=Auto  DifferentiatorICPrevScaledInput=0  DifferentiatorOutMin=[]  DifferentiatorOutMax=[]  InitialConditionSetting=State (most efficient)  FilterDiffOutCoefMin=[]  FilterDiffOutCoefMax=[]  SumDenOutMin=[]  SumDenOutMax=[]  SumNumOutMin=[]  SumNumOutMax=[]  ReciprocalOutMin=[]  ReciprocalOutMax=[]  DivideOutMin=[]  DivideOutMax=[]  TunerSelectOption=Transfer Function Based (PID Tuner App)
  Scope : Scope
  Scope1 : Scope  NumInputPorts=2
  Subsystem : Subsystem
  Sum2 : Sum  Inputs=|+-
  F_tractionDemand_N : Outport
  wires:
  v_drivingCycle_m/s/1 -> Sum2/1
  Sum2/1 -> PID Controller1/1
  PID Controller1/1 -> Scope/1, MATLAB Function/1(pid)
  MATLAB Function/1(s) -> Subsystem/1(F_soll), Scope1/1  "F_soll"
  Subsystem/1(Out1) -> F_tractionDemand_N/1, Scope1/2  "F_actual"
  v_train/1 -> Subsystem/2(v_train_ist), Sum2/2

== system xEMU_SimulationModel3_rule1/Train Dynamics (TRM)/Variant Subsystem/v_t_model/Driving Resistances ==
  v_train : Inport
  gradient : Inport  Port=2
  total mass : Inport  Port=3
  Add : Sum  Inputs=-+
  Constant1 : Constant  Value=atan(ENV.height.Height(end)/ENV.height.position(end))
  Gain : Gain  Gain=g_drt
  Gain1 : Gain  Gain=0.0015
  Gain2 : Gain  Gain=1/1000*3.6*0.025
  MATLAB Function1 : MATLAB Function  TreatAsAtomicUnit=on
  Product{,1..3} (4 alike) : Product
  Scope : Scope
  Scope2 : Scope
  Subtract : Sum  Inputs=++++
  Trigonometric Function : Trigonometry
  Trigonometric Function1 : Trigonometry
  Trigonometric Function2 : Trigonometry  Operator=cos
  air resistance : Fcn  Expr=Cw_tdn_abs*A_tdn_m2*(PI_tdn/2)*(u)^2
  air&gradient_resistance_N : Outport
  tag scope: gradient=global
  wires:
  Product3/1 -> Scope2/1, Add/2
  Product1/1 -> Gain2/1
  Trigonometric Function1/1 -> Product3/2
  Product/1 -> Add/1, Subtract/3
  MATLAB Function1/1(Froll) -> Subtract/4
  v_train/1 -> Product1/1, MATLAB Function1/1(v), air resistance/1
  Product2/1 -> MATLAB Function1/2(froll)
  Gain/1 -> Product3/1, Gain1/1, Product/2
  Add/1 -> Scope/1, [gradient]
  gradient/1 -> Trigonometric Function2/1, Trigonometric Function/1
  Subtract/1 -> air&gradient_resistance_N/1
  Trigonometric Function/1 -> Product/1
  air resistance/1 -> Subtract/2
  Gain1/1 -> Product2/1
  Gain2/1 -> Subtract/1
  Trigonometric Function2/1 -> Product2/2
  total mass/1 -> Product1/2, Gain/1
  Constant1/1 -> Trigonometric Function1/1

== system xEMU_SimulationModel3_rule1/Train Dynamics (TRM)/Variant Subsystem/v_t_model/Train Longitudinal Dynamics ==
  note: a
  air&gradient_resistance_N : Inport
  n_passengers_abs : Inport  Port=2
  F_traction_N : Inport  Port=3
  Constant : Constant  Value=m_train_tdn_kg
  Divide : Product  Inputs=/*
  Gain : Gain  Gain=m_passenger_tdn_kg
  Integrator : Integrator  LimitOutput=on  LowerSaturationLimit=0
  Subtract : Sum
  Sum : Sum  Inputs=-+|
  total_mass_kg : Outport
  v_train_m/s : Outport  Port=2
  wires:
  air&gradient_resistance_N/1 -> Sum/1
  Integrator/1 -> v_train_m/s/1  "v"
  Sum/1 -> Divide/2
  n_passengers_abs/1 -> Gain/1
  Constant/1 -> Subtract/2
  Gain/1 -> Subtract/1
  F_traction_N/1 -> Sum/2
  Divide/1 -> Integrator/1  "a"
  Subtract/1 -> Divide/1, total_mass_kg/1

== system xEMU_SimulationModel3_rule1/Battery (BAT)_komplex/Subsystem/ElectricalCircuit/Cellelement_Elem1/OhmicResistance_Elem1 ==
  T : Inport
  SoC : Inport  Port=2
  Object : Lookup_n-D  BreakpointsForDimension1=[10 25 35 45]  BreakpointsForDimension2=[0 5 10 15 20 25 30 35 40 45 50 55 60 65 70 75 80 85 90 95 100]  Table=[0.000771968526803023 0.000748369146052688 0.000724881421092217 0.000703132225685812 0.000681405509074902 0.000662730818510104 0.000645251487485153 0.000631118585145968 0.000617074401605558 0.000603444604710944 0.000588975057934144 0.000574938504017678 0.000557784934803898 0.00054413410139131 0.0005282009160006 0.000513150140111006 0.000497368589356565 0.000480432670706108 0.000468327505260267 0.000459151981966271 0.00044721979103073;0.000607538709252138 0.000591906678896865 0.000579251526535265 0.000566736941111578 0.000554267843362006 0.00054193499054528 0.000528289326909059 0.000518627966086254 0.000508454014080012 0.000498619432440266 0.000487314814733121 0.000479311632434861 0.000469030628019127 0.000460272639433147 0.000450192255124041 0.000439297274666459 0.000428239996856566 0.000417728515462718 0.000409674349230244 0.000404459083809335 0.000392103511229194;0.000532360065388155 0.00052360448028229 0.000514747341431657 0.000504947167518555 0.00049503906759317 0.000486377259235303 0.000477750186118738 0.000468937804866539 0.000461447107731537 0.000454666596698088 0.000447908076851307 0.000441183098574019 0.000431588050586221 0.000424993386722809 0.000419393984065282 0.000411618970605753 0.000403616676362054 0.000395831770376174 0.000387955856358833 0.000382048896042462 0.000377611755738171;0.000491068260475341 0.00048241524334078 0.000478893043251579 0.000474231745067159 0.000463419524146351 0.000453533482441388 0.000448154117766324 0.000444198582958616 0.000440406492727549 0.000434596688885989 0.000428993938540256 0.000423688723613095 0.000417260659200824 0.000411063362411327 0.000403315228447255 0.00040014675568242 0.000393272441695337 0.00038814268028836 0.00038290705375794 0.000373250570942629 0.000364317930560238]  ExtrapMethod=Clip  RndMeth=Simplest  InputSameDT=on
  tag scope: ID1_ObjR=global
  wires:
  Object/1 -> [ID1_ObjR]
  T/1 -> Object/1
  SoC/1 -> Object/2

== system xEMU_SimulationModel3_rule1/Battery (BAT)_komplex/Subsystem/ElectricalCircuit/Cellelement_Elem1/ParallelRC_Elem5 ==
  T : Inport
  SoC : Inport  Port=2
  Object : Lookup_n-D  BreakpointsForDimension1=[10 25 35 45]  BreakpointsForDimension2=[0 5 10 15 20 25 30 35 40 45 50 55 60 65 70 75 80 85 90 95 100]  Table=[0.00764728927709652 0.00474423865923742 0.00203396840695321 0.00231038728921286 0.00206615832855233 0.00190458593231064 0.00185856156152465 0.00165198805708657 0.00171477833745534 0.00153065139517468 0.00163818950613008 0.00153651551312183 0.000909011357916661 0.00118776928802931 0.00170773809968292 0.00152798511163003 0.00132357118315589 0.00119016648121892 0.000863319393777177 0.0011826590260031 0.00118270083620402;0.00587553867538804 0.00154839875781604 0.00145455635275654 0.00108066337379952 0.00123647187367758 0.00134505637092348 0.00119010790610603 0.000914840836507952 0.00120902316731515 0.00106177386040427 0.00113510439044689 0.00109305083615692 0.000947546726337524 0.00125215588006856 0.00102142196697215 0.000978919305729693 0.000925383538786521 0.000739308136109667 0.000689063876872616 0.000876876834715341 0.000876880431629726;0.00139386150279849 0.00145440718530885 0.00123686321307858 0.00106972733310903 0.000902712396975044 0.000963263486504002 0.000980885342233891 0.000671712100771071 0.000985515464118976 0.000801732026212843 0.000860489547883767 0.00083824337824724 0.00101406228045639 0.000968508887655047 0.000777585656833542 0.000634467307635599 0.000508360442881214 0.000537670622708236 0.000275193202810073 0.000269396711698707 0.00026940006710819;0.000860744687168582 0.00104628594847602 0.000964774286317786 0.000903956546944867 0.0008883571130244 0.000798285384222583 0.0006483394565504 0.000535561389178171 0.000508091265821407 0.00044910739208783 0.000400866304532207 0.000417700255613791 0.00064414451482694 0.000568643085179211 0.000398699574906687 0.000347961616179267 0.000331212768477187 0.000230954269983984 0.000305644439156634 0.000129027087395457 0.000128998271017311]  ExtrapMethod=Clip  RndMeth=Simplest  InputSameDT=on
  Tau : Lookup_n-D  BreakpointsForDimension1=[10 25 35 45]  BreakpointsForDimension2=[0 5 10 15 20 25 30 35 40 45 50 55 60 65 70 75 80 85 90 95 100]  Table=[22.1898909514035 26.5842152221479 31.7411994240462 47.8251884127405 47.8565404302297 47.422670108927 51.740171298322 46.2462097099599 48.3835662371059 44.7822763601721 43.1857659402676 42.4016771471478 24.3581391906999 28.5703136670354 44.416902537374 37.3094150990016 35.3769956666779 35.4705039135581 39.8139799767232 33.3061522268275 33.30599689333;22.0049861740439 25.0221638317897 37.7189952817354 22.6587659796224 37.1615499291492 37.6703675362051 36.2787721869487 22.2875536653091 33.2265829072705 32.8555058583998 30.9807312625166 32.7305073519293 25.5650300629843 32.233048150971 25.7482720766016 26.5721540946532 25.0756848266839 26.9317784085936 24.9760975672177 24.4770988013198 24.4769865270928;21.3780024298734 32.1910645264531 35.0394493423987 33.5400382823725 29.184625958329 32.1928242068211 29.675228194561 17.74604903142 27.7270396338011 28.6090915478394 28.5868733209495 31.9498489317353 27.9848660278726 23.3533871912033 21.3971772880622 21.6270074341763 21.1486235390482 19.9929459827115 7.48768361844528 20.985018857628 20.9849996151504;15.238189698917 36.0034225048109 30.755391417161 28.529975322527 26.1807246599539 26.7135294207742 18.3293756250247 14.0981192102909 12.1591957639524 11.8539599745503 10.0876535743557 9.92575052180348 15.4595077908202 10.0151490899665 8.45913947036717 8.43707343464333 12.3511967627153 7.90200149673811 13.3035597189383 9.99100957924203 9.99099938855902]  ExtrapMethod=Clip  RndMeth=Simplest  InputSameDT=on
  tag scope: ID2_ObjR=global, ID2_ObjTau=global
  wires:
  Object/1 -> [ID2_ObjR]
  T/1 -> Object/1, Tau/1
  SoC/1 -> Object/2, Tau/2
  Tau/1 -> [ID2_ObjTau]

== system xEMU_SimulationModel3_rule1/Battery (BAT)_komplex/Subsystem/ElectricalCircuit/Cellelement_Elem1/ParallelRC_Elem6 ==
  T : Inport
  SoC : Inport  Port=2
  Object : Lookup_n-D  BreakpointsForDimension1=[10 25 35 45]  BreakpointsForDimension2=[0 5 10 15 20 25 30 35 40 45 50 55 60 65 70 75 80 85 90 95 100]  Table=[0.00612505138589157 0.00407283419232278 0.00211029694509598 0.00158426234016647 0.00154050558572137 0.00135695046447579 0.00174483106257212 0.00128267385631804 0.0015888070219515 0.00145042307444027 0.00189788894173659 0.00191806538662505 0.00252122095787405 0.00178546502838825 0.00069277294068049 0.000722858269843324 0.000687448865120982 0.000713033101262336 0.000765267477319311 0.000747209485853623 0.000747210010492783;0.0028803728228227 0.00166494478241037 0.00130679609125278 0.0014088956332448 0.00100702693562222 0.00098864172422517 0.00111459557282459 0.00102368360719172 0.000893755458255841 0.000915978165021569 0.000912913896198892 0.000927851930931685 0.0006587861100766 0.000565769571977714 0.000430224974782173 0.000596297603341754 0.000638377058612318 0.000640779681863622 0.000475648188476712 0.000644113634046433 0.000644109504448214;0.00160384570742686 0.000803193890546296 0.00117020815660094 0.000822719732794618 0.000820848778809978 0.000745228772184654 0.000521027261974307 0.000675990896562611 0.0006374826532219 0.000809498752713429 0.00075344471045016 0.000777186513743439 0.000583235753089049 0.000461271319101388 0.000264239208753733 0.000315200624621732 0.000385153057603513 0.000355119347985819 0.000466231518822687 0.000385143980736301 0.000385139918760484;0.0011058837581201 0.00102327958142904 0.000854017589770261 0.000620354722485578 0.000533612297837053 0.000554932892670066 0.000545949328641521 0.000564765991762031 0.000557954507833749 0.000571334206155164 0.000611361350603188 0.000581992936132193 0.00032553522338182 0.000308453864003534 0.000245402536897638 0.000267237748104272 0.000271149225568223 0.000321983778533294 0.000321857571242993 0.000302892217354013 -1.93335457885538e-05]  ExtrapMethod=Clip  RndMeth=Simplest  InputSameDT=on
  Tau : Lookup_n-D  BreakpointsForDimension1=[10 25 35 45]  BreakpointsForDimension2=[0 5 10 15 20 25 30 35 40 45 50 55 60 65 70 75 80 85 90 95 100]  Table=[8894.04992458898 5583.22117357318 2395.80166283633 1222.27613662254 1292.01428487515 1131.61950126611 1623.83618664477 1094.67312849281 1491.82790066986 1278.05994799138 1511.7809635949 1129.87245676405 1286.93745584224 307.608419371418 476.725699330865 817.638115923972 835.62971341781 897.870159627786 1027.24664256503 940.219265730565 940.220014985091;1666.19698223227 1725.30031527279 1412.44748834952 2019.88206707202 1154.54617101241 1184.41979676773 1449.16341083556 1620.94357186667 1045.1208926029 1004.12263417972 914.704129892067 953.590993454473 855.556450253306 315.371820985523 764.232111251126 1212.1035795243 1203.87532778525 1113.94605881351 799.434252905741 1183.94384406215 1183.89402126425;1589.88514034659 650.112197316073 1467.02952638775 1041.69496288167 1117.68067213788 1010.25387619464 687.13401580774 1275.80911085289 922.171131504742 1156.04494477055 1056.70609053138 1154.31370451518 378.605742790933 794.666924710376 608.839146423894 734.769709561691 837.435325614985 712.905447599833 1042.2052053285 772.554093207652 772.54991646515;1621.53825009247 1313.72871612921 1200.47636507688 907.632286442718 757.517098195639 888.555824764039 1015.72794287654 1295.65572744615 1196.63571128977 1146.57640266193 1207.77397098176 1351.13029871221 1179.47682188115 795.706769335172 829.656008403581 808.642698694274 744.407212202976 855.955983164718 745.60016510757 845.668870041818 2073.68071042286]  ExtrapMethod=Clip  RndMeth=Simplest  InputSameDT=on
  tag scope: ID3_ObjR=global, ID3_ObjTau=global
  wires:
  Object/1 -> [ID3_ObjR]
  T/1 -> Object/1, Tau/1
  SoC/1 -> Object/2, Tau/2
  Tau/1 -> [ID3_ObjTau]
